simulink model "MomentForceCBAgent"  (Simulink 6.2)
settings: Solver=ode45  SolverMode=SingleTasking  StartTime=0.0  StopTime=10.0  RelTol=1e-3  AbsTol=1e-6
settings Model: Creator=The MathWorks Inc.  LastModifiedBy=suarezjl  ExtModeTrigMode=oneshot  ExtModeArmWhenConnect=off  ExtModeAutoUpdateStatusClock=off
settings DataIOCC: LimitDataPoints=off  SignalLoggingName=logsOut
settings OptimizationCC: BooleanDataType=off  InlineInvariantSignals=on
settings DebuggingCC: CheckExecutionContextPreStartOutputMsg=on  CheckExecutionContextRuntimeOutputMsg=on  IntegerOverflowMsg=none
settings HardwareCC: TargetUnknown=on
settings ModelReferenceCC: UpdateModelReferenceTargets=IfOutOfDate

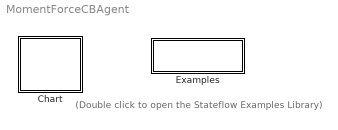
== system MomentForceCBAgent ==
  note: (Double click to open the
      | Stateflow Examples Library)
  Chart : Stateflow chart
  Examples : Subsystem
      settings: OpenFcn=sf('Private','sf_examples')
      mask Display: disp('Examples')

== system MomentForceCBAgent/Examples ==

== stateflow chart Chart ==
  state Initialize
    Aquateen\ControlBasisModule\ForceSensor\StateMachine.LoadSM()
    Aquateen\ControlBasisModule\ForceSensor\StateMachine.Start()
    Aquateen\ControlBasisModule\HP3JCAgent\HP3JC.connect_Initialize()
    Aquateen\ControlBasisModule\HP3JCAgent\HP3JC.servo_ServoOn()
    Aquateen\ControlBasisModule\HP3JCAgent\HP3JC.read_CurrentPosition()
    Aquateen\ControlBasisModule\MomentForceCB\MomentForceCB.Initialize()
  state ReadPosition
    Aquateen\ControlBasisModule\HP3JCAgent\HP3JC.read_CurrentPosition()
    Aquateen\ControlBasisModule\MomentForceCB\MomentForceCB.ComputeControlBasis()
    Aquateen\ControlBasisModule\HP3JCAgent\HP3JC.move_JointAngles()
  state \Stop
    Aquateen\ControlBasisModule\ForceSensor\StateMachine.Stop()
    Aquateen\ControlBasisModule\HP3JCAgent\HP3JC.error_ClearError()
    Aquateen\ControlBasisModule\HP3JCAgent\HP3JC.error_ClearAlarm()
    Aquateen\ControlBasisModule\HP3JCAgent\HP3JC.job_SelectJob()
    Aquateen\ControlBasisModule\HP3JCAgent\HP3JC.job_StartJob()
    Aquateen\ControlBasisModule\MomentForceCB\StateMachine.Wait(500)
    Aquateen\ControlBasisModule\HP3JCAgent\HP3JC.connect_Disconnect()
  (default) -> Initialize : Start
  Initialize -> ReadPosition : Always
  ReadPosition -> ReadPosition [order 1] : Default
  ReadPosition -> \Stop [order 2] : Signal="End"
